simulink model "simulation of opendata "  (R2024b)
settings: Solver=ode4  StartTime=0.0  StopTime=10  FixedStep=0.0001  RelTol=1e-3
settings Model: Creator=adm  LastModifiedBy=adm

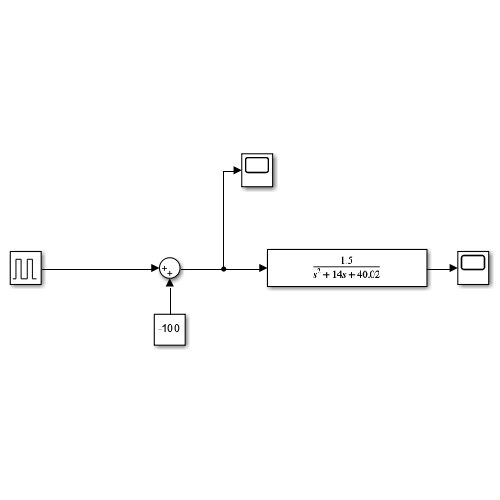
[thumbnail: Simulink's stored preview of the top-level diagram]
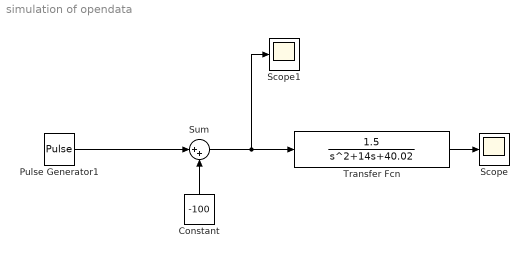
== system simulation of opendata  ==
  Constant : Constant  Value=-100
  Pulse Generator1 : DiscretePulseGenerator  PulseType=Time based  Amplitude=200  Period=10  PulseWidth=50
  Scope : Scope
  Scope1 : Scope
  Sum : Sum  Inputs=|++
  Transfer Fcn : TransferFcn  Numerator=[1.5]  Denominator=[1 14 40.02]
  wires:
  Transfer Fcn/1 -> Scope/1
  Sum/1 -> Scope1/1, Transfer Fcn/1
  Pulse Generator1/1 -> Sum/1
  Constant/1 -> Sum/2
